simulink model "AccPed_DrvDemStpLim"  (R2016b)
settings: configuration reference "CodeGenConfigSet" (kept outside this file)
values from neighbouring files (symbols this model uses):
  AccPed_dnMaxRmp_C = Calibration.Parameter    [init_AccPed_DrvDemStpLim.m]    (also in init_AccPed_DrvDemStpLim_SIL.m = Simulink.Parameter)
  AccPed_dtrqDwnLim_MAP = Calibration.Parameter    [init_AccPed_DrvDemStpLim.m]    (also in init_AccPed_DrvDemStpLim_SIL.m = Simulink.Parameter)
  AccPed_dtrqDwnLim_MAPX = Calibration.Parameter    [init_AccPed_DrvDemStpLim.m]    (also in init_AccPed_DrvDemStpLim_SIL.m = Simulink.Parameter)
  AccPed_dtrqDwnLim_MAPY = Calibration.Parameter    [init_AccPed_DrvDemStpLim.m]    (also in init_AccPed_DrvDemStpLim_SIL.m = Simulink.Parameter)
  AccPed_dtrqUpLim_MAP = Calibration.Parameter    [init_AccPed_DrvDemStpLim.m]    (also in init_AccPed_DrvDemStpLim_SIL.m = Simulink.Parameter)
  AccPed_dtrqUpLim_MAPX = Calibration.Parameter    [init_AccPed_DrvDemStpLim.m]    (also in init_AccPed_DrvDemStpLim_SIL.m = Simulink.Parameter)
  AccPed_dtrqUpLim_MAPY = Calibration.Parameter    [init_AccPed_DrvDemStpLim.m]    (also in init_AccPed_DrvDemStpLim_SIL.m = Simulink.Parameter)
  AccPed_nMaxRmp_C = Calibration.Parameter    [init_AccPed_DrvDemStpLim.m]    (also in init_AccPed_DrvDemStpLim_SIL.m = Simulink.Parameter)
  AccPed_swtStpLim_C = Calibration.Parameter    [init_AccPed_DrvDemStpLim.m]    (also in init_AccPed_DrvDemStpLim_SIL.m = Simulink.Parameter)
  TRQ_ZERO = int16(0)    [init_AccPed_DrvDemStpLim.m]    (also in init_AccPed_DrvDemStpLim_SIL.m)
undefined symbols (not defined in the file or in its folder): AccPed_DrvDemStpLim_DT, Switch_conv
libraries: CXLib x3, simulink x1
settings Model: Creator=lenovo  LastModifiedBy=wangrui
settings ConfigSetRef: SourceLocation=Base Workspace

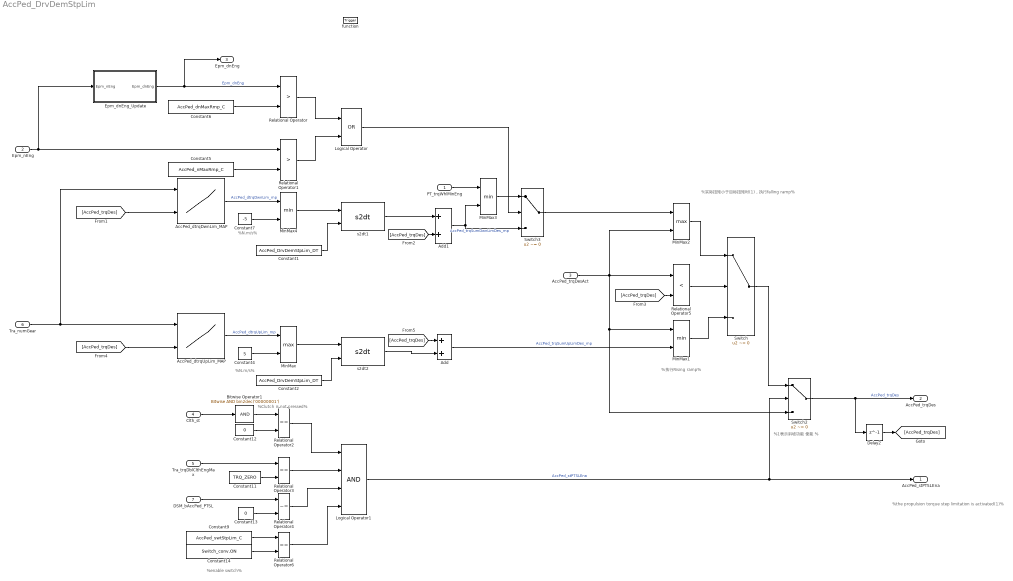
== system AccPed_DrvDemStpLim ==
  note: %执行Rising ramp%
  note: %N.m/s%
  note: %the propulsion torque step limitation is activated(1)%
  note: %Clutch is not pressed%
  note: %enable switch%
  note: %实际扭矩小于目标扭矩时(1)，执行falling ramp%
  note: %N.m/s%
  note: %1表示斜坡功能 使能 %
  PT_trqWhlMinEng : Inport  Tag=Nm  Description=Minimum wheel torque from the engine  OutMin=-3000  OutMax=3000  OutDataTypeStr=Trq_Nm
  Epm_nEng : Inport  Tag=rpm  Description=Engine speed  Port=2  OutMin=0  OutMax=6000  OutDataTypeStr=EngSpeed_rpm
  AccPed_trqDesAct : Inport  Tag=Nm  Description=driver torque raw of propulsion  Port=3  OutMin=-3000  OutMax=3000  OutDataTypeStr=Trq_Nm
  Clth_st : Inport  Description=Clutch information  Port=4  OutMin=0  OutMax=255  OutDataTypeStr=State_uint8
  Tra_trqDblClthEngMax : Inport  Tag=Nm  Description=Application parameter for minimum torque of systemdegratation Nm  Port=5  OutMin=-3000  OutMax=3000  OutDataTypeStr=Trq_Nm
  Tra_numGear : Inport  Description=Current gear information  Port=6  OutMin=-128  OutMax=127  OutDataTypeStr=Tra_num
  DSM_bAccPed_PTSL : Inport  Description=status of FId_AccPed_PTSL  Port=7  OutMin=0  OutMax=1  OutDataTypeStr=boolean
  function : TriggerPort  TriggerType=function-call  VariantControl=Variant
  " AccPed_dtrqDwnLim_MAP" : Lookup_n-D  BreakpointsForDimension1=AccPed_dtrqDwnLim_MAPY  BreakpointsForDimension2=AccPed_dtrqDwnLim_MAPX  IndexSearchMethod=Linear search  BeginIndexSearchUsingPreviousIndexResult=on  Table=AccPed_dtrqDwnLim_MAP  ExtrapMethod=Clip  UseLastTableValue=on  InternalRulePriority=Speed  OutDataTypeStr=Inherit: Inherit via back propagation  SaturateOnIntegerOverflow=on
  " AccPed_dtrqUpLim_MAP" : Lookup_n-D  BreakpointsForDimension1=AccPed_dtrqUpLim_MAPY  BreakpointsForDimension2=AccPed_dtrqUpLim_MAPX  IndexSearchMethod=Linear search  BeginIndexSearchUsingPreviousIndexResult=on  Table=AccPed_dtrqUpLim_MAP  ExtrapMethod=Clip  UseLastTableValue=on  InternalRulePriority=Speed  OutDataTypeStr=Inherit: Inherit via back propagation  SaturateOnIntegerOverflow=on
  Add : Sum  OutDataTypeStr=Inherit: Inherit via back propagation  SaturateOnIntegerOverflow=on  InputSameDT=on
  Add1 : Sum  OutDataTypeStr=Inherit: Inherit via back propagation  SaturateOnIntegerOverflow=on  InputSameDT=on
  Bitwise Operator1 : simulink/Logic and Bit Operations/Bitwise Operator  logicop=AND  UseBitMask=on  BitMask=bin2dec('00000001')  BitMaskRealWorld=Stored Integer
  Constant1 : Constant  Value=AccPed_DrvDemStpLim_DT
  Constant11 : Constant  Value=TRQ_ZERO  OutDataTypeStr=Trq_Nm
  Constant12 : Constant  Value=0  OutDataTypeStr=uint8
  Constant13 : Constant  Value=0  OutDataTypeStr=Inherit: Inherit via back propagation
  Constant14 : Constant  Value=Switch_conv.ON  OutDataTypeStr=Inherit: Inherit via back propagation
  Constant2 : Constant  Value=AccPed_DrvDemStpLim_DT
  Constant4 : Constant  Value=5  OutDataTypeStr=Inherit: Inherit via back propagation
  Constant5 : Constant  Value=AccPed_nMaxRmp_C
  Constant6 : Constant  Value=AccPed_dnMaxRmp_C
  Constant7 : Constant  Value=-5  OutDataTypeStr=Inherit: Inherit via back propagation
  Constant9 : Constant  Value=AccPed_swtStpLim_C
  Delay2 : Delay  DelayLength=1  InitialCondition=0
  Epm_dnEng_Update : Subsystem
  Logical Operator : Logic  Operator=OR  OutDataTypeStr=boolean
  Logical Operator1 : Logic  Inputs=4  OutDataTypeStr=boolean
  MinMax : MinMax  Function=max  Inputs=2  InputSameDT=on
  MinMax1 : MinMax  Inputs=2  InputSameDT=on
  MinMax2 : MinMax  Function=max  Inputs=2  InputSameDT=on
  MinMax3 : MinMax  Inputs=2  InputSameDT=on
  MinMax4 : MinMax  Inputs=2  InputSameDT=on
  Relational Operator : RelationalOperator  Operator=>  OutDataTypeStr=boolean  RndMeth=Simplest  InputSameDT=on
  Relational Operator1 : RelationalOperator  Operator=>  OutDataTypeStr=boolean  RndMeth=Simplest  InputSameDT=on
  Relational Operator2 : RelationalOperator  Operator===  OutDataTypeStr=boolean  RndMeth=Simplest  InputSameDT=on
  Relational Operator3 : RelationalOperator  Operator===  OutDataTypeStr=boolean  RndMeth=Simplest  InputSameDT=on
  Relational Operator4 : RelationalOperator  Operator=~=  OutDataTypeStr=boolean  RndMeth=Simplest  InputSameDT=on
  Relational Operator5 : RelationalOperator  Operator=<  OutDataTypeStr=boolean  RndMeth=Simplest  InputSameDT=on
  Relational Operator6 : RelationalOperator  Operator===  OutDataTypeStr=boolean  RndMeth=Simplest  InputSameDT=on
  Switch : Switch  Criteria=u2 ~= 0  InputSameDT=on
  Switch2 : Switch  Criteria=u2 ~= 0  InputSameDT=on
  Switch3 : Switch  Criteria=u2 ~= 0  InputSameDT=on
  s2dt1 : CXLib/s2dt
  s2dt2 : CXLib/s2dt
  AccPed_stPTSLEna : Outport  Description=Enable status of the propulsion torque step limitation  OutMin=0  OutMax=1  OutDataTypeStr=boolean
  AccPed_trqDes : Outport  Tag=Nm  Description=Driver torque value of propulsion after step limitation  Port=2  OutMin=-3000  OutMax=3000  OutDataTypeStr=Trq_Nm
  Epm_dnEng : Outport  Tag=rpm/s  Description=Engine speed gradient calculated over current crankshaft-segment (S0-S0 or S1-S1)  Port=3  OutMin=-12000  OutMax=12000  OutDataTypeStr=EngSpeed_rpm_s
  wires:
  s2dt2/1 -> Add/2
  MinMax/1 -> s2dt2/1
  [AccPed_trqDes] -> Add/1
  [AccPed_trqDes] -> " AccPed_dtrqUpLim_MAP"/2
  [AccPed_trqDes] -> Relational Operator5/2
  [AccPed_trqDes] -> " AccPed_dtrqDwnLim_MAP"/2
  [AccPed_trqDes] -> Add1/2
  Delay2/1 -> [AccPed_trqDes]
  Tra_numGear/1 -> " AccPed_dtrqUpLim_MAP"/1, " AccPed_dtrqDwnLim_MAP"/1
  " AccPed_dtrqUpLim_MAP"/1 -> MinMax/1  "AccPed_dtrqUpLim_mp"
  Constant4/1 -> MinMax/2
  Add/1 -> MinMax1/2  "AccPed_trqSumUpLimDes_mp"
  AccPed_trqDesAct/1 -> MinMax1/1, Switch2/3, Relational Operator5/1, MinMax2/2
  MinMax2/1 -> Switch/1
  MinMax1/1 -> Switch/3
  Epm_dnEng_Update/1(Epm_dnEng) -> Epm_dnEng/1, Relational Operator/1  "Epm_dnEng"
  Constant6/1 -> Relational Operator/2
  Constant5/1 -> Relational Operator1/2
  Epm_nEng/1 -> Relational Operator1/1, Epm_dnEng_Update/1(Epm_nEng)
  Relational Operator/1 -> Logical Operator/1
  Relational Operator1/1 -> Logical Operator/2
  " AccPed_dtrqDwnLim_MAP"/1 -> MinMax4/1  "AccPed_dtrqDwnLim_mp"
  Constant7/1 -> MinMax4/2
  MinMax4/1 -> s2dt1/1
  Constant1/1 -> s2dt1/2
  s2dt1/1 -> Add1/1
  Switch/1 -> Switch2/1
  Switch2/1 -> AccPed_trqDes/1, Delay2/1  "AccPed_trqDes"
  Add1/1 -> Switch3/3, MinMax3/2  "AccPed_trqSumDwnLimDes_mp"
  PT_trqWhlMinEng/1 -> MinMax3/1
  MinMax3/1 -> Switch3/1
  Logical Operator/1 -> Switch3/2
  Switch3/1 -> MinMax2/1
  Relational Operator2/1 -> Logical Operator1/1
  Relational Operator3/1 -> Logical Operator1/2
  Tra_trqDblClthEngMax/1 -> Relational Operator3/1
  Constant11/1 -> Relational Operator3/2
  Constant12/1 -> Relational Operator2/2
  Logical Operator1/1 -> AccPed_stPTSLEna/1, Switch2/2  "AccPed_stPTSLEna"
  DSM_bAccPed_PTSL/1 -> Relational Operator4/1
  Constant13/1 -> Relational Operator4/2
  Relational Operator4/1 -> Logical Operator1/3
  Clth_st/1 -> Bitwise Operator1/1
  Bitwise Operator1/1 -> Relational Operator2/1
  Relational Operator5/1 -> Switch/2
  Constant9/1 -> Relational Operator6/1
  Constant14/1 -> Relational Operator6/2
  Relational Operator6/1 -> Logical Operator1/4
  Constant2/1 -> s2dt2/2

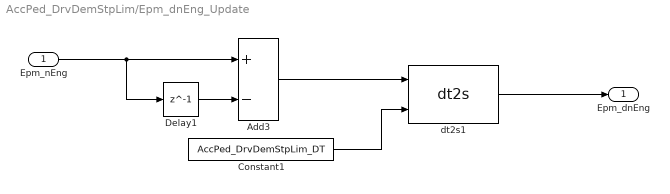
== system AccPed_DrvDemStpLim/Epm_dnEng_Update ==
  Epm_nEng : Inport
  Add3 : Sum  Inputs=+-  OutDataTypeStr=Inherit: Inherit via back propagation  SaturateOnIntegerOverflow=on  InputSameDT=on
  Constant1 : Constant  Value=AccPed_DrvDemStpLim_DT  OutDataTypeStr=Inherit: Inherit via back propagation
  Delay1 : Delay  DelayLength=1  InitialCondition=0
  dt2s1 : CXLib/dt2s
  Epm_dnEng : Outport
  wires:
  Add3/1 -> dt2s1/1
  Epm_nEng/1 -> Add3/1, Delay1/1
  Delay1/1 -> Add3/2
  dt2s1/1 -> Epm_dnEng/1
  Constant1/1 -> dt2s1/2
